simulink model "ai_optimal_path_depth_v2_4_g100"  (R2020a)
settings: Solver=FixedStepDiscrete  StartTime=0.0  StopTime=inf  FixedStep=0.2  RelTol=1e-3  EnableMultiTasking=on
model workspace (MAT data in the model file):
  SL_ROS_VariableLengthArrays_MaxSizes : object (value not decoded)
undefined symbols (not defined in the file): Data, Data_SL_Info
libraries: robotlib x33
(part 2 of 2)

== matlab function ai_optimal_path_depth_v2_4_g100/MATLAB Function ==
  data: current_pos input; point input; distance input; bboxes_front_raw input; bboxes_back_raw input; bboxes_left_raw input; bboxes_right_raw input; openpoint_front output; image_size input; image_grid input; openpoint_back output; openpoint_left output; openpoint_right output; count output; obstacle_check output
function [openpoint_front,openpoint_back,openpoint_left,openpoint_right,count,obstacle_check] = fcn(current_pos,point,distance,bboxes_front_raw,bboxes_back_raw,bboxes_left_raw,bboxes_right_raw,image_size,image_grid)
% function [distance_ref_front,distance_ref_back,distance_ref_left,distance_ref_right] = fcn(point,I_front_rgb,I_back_rgb,I_left_rgb,I_right_rgb,bboxes_front_raw,bboxes_back_raw,bboxes_left_raw,bboxes_right_raw)
% image_grid = 0.05;

% pos_x = current_pos(1);
% pos_y = current_pos(2);
% pos_z = current_pos(3);
% pos_x = current_pos.Poses(end).Pose.Position.X;
% pos_y = current_pos.Poses(end).Pose.Position.Y;
% pos_z = current_pos.Poses(end).Pose.Position.Z;

pos_x = current_pos.Pose.Pose.Position.X;
pos_y = current_pos.Pose.Pose.Position.Y;
pos_z = current_pos.Pose.Pose.Position.Z;
% image_size = 500;
% image_size = I_front_rgb(:,:,1);
% image_size = I_back_rgb(:,:,1);
% image_size = I_left_rgb(:,:,1);
% image_size = I_right_rgb(:,:,1);

openpoint_front = nan(5,6);
openpoint_back = nan(5,6);
openpoint_left = nan(5,6);
openpoint_right = nan(5,6);
count = zeros(5,4);
obstacle_check = zeros(5,4);
thickness = distance/2;
% thickness = 2;
obstacle_safety = 0.3;

% bboxes_front = int16(bboxes_front_raw);
% bboxes_back = int16(bboxes_back_raw);
% bboxes_left = int16(bboxes_left_raw);
% bboxes_right = int16(bboxes_right_raw);
% bboxes_front = reshape(int16(bboxes_front_raw),[5, 4]);
% bboxes_back = reshape(int16(bboxes_back_raw),[5, 4]);
% bboxes_left = reshape(int16(bboxes_left_raw),[5, 4]);
% bboxes_right = reshape(int16(bboxes_right_raw),[5, 4]);

bboxes_front = nan(5,4);
bboxes_back = nan(5,4);
bboxes_left = nan(5,4);
bboxes_right = nan(5,4);
for ttt = 1:4
    for sss = 1:5
        bboxes_front(sss,ttt) = int16(bboxes_front_raw(5*(ttt-1)+sss));
        bboxes_back(sss,ttt) = int16(bboxes_back_raw(5*(ttt-1)+sss));
        bboxes_left(sss,ttt) = int16(bboxes_left_raw(5*(ttt-1)+sss));
        bboxes_right(sss,ttt) = int16(bboxes_right_raw(5*(ttt-1)+sss));
    end
end
        
% distance_ref_front=[];
% distance_ref_back=[];
% distance_ref_left=[];
% distance_ref_right=[];

distance_ref_front=nan(5,1);
distance_ref_back=nan(5,1);
distance_ref_left=nan(5,1);
distance_ref_right=nan(5,1);

% aaa=1;
% if ~isempty(bboxes_front)
if ~sum(bboxes_front)==0
    for aaa = 1:numel(nonzeros(bboxes_front))/4
        if (bboxes_front(aaa,1)+bboxes_front(aaa,3)/2) >= (image_size)/2
            distance_ref_front(aaa) = bboxes_front(aaa,1)+bboxes_front(aaa,3);
        else
            distance_ref_front(aaa) = bboxes_front(aaa,1);
        end
    end
    distance_ref_front= -(distance_ref_front - (image_size)/2)*image_grid;           % 醫뚰몴媛?(m)
end

% if ~isempty(bboxes_back)
if ~sum(bboxes_back)==0
    for aaa = 1:numel(nonzeros(bboxes_back))/4
        if (bboxes_back(aaa,1)+bboxes_back(aaa,3)/2) >= (image_size)/2
            distance_ref_back(aaa) = bboxes_back(aaa,1)+bboxes_back(aaa,3);
        else
            distance_ref_back(aaa) = bboxes_back(aaa,1);
        end
    end
    distance_ref_back= -(distance_ref_back - (image_size)/2)*image_grid;              % 醫뚰몴媛?(m)
end

% if ~isempty(bboxes_left)
if ~sum(bboxes_left)==0
    for aaa = 1:numel(nonzeros(bboxes_left))/4
        if (bboxes_left(aaa,1)+bboxes_left(aaa,3)/2) >= (image_size)/2
            distance_ref_left(aaa) = bboxes_left(aaa,1)+bboxes_left(aaa,3);
        else
            distance_ref_left(aaa) = bboxes_left(aaa,1);
        end
    end
    distance_ref_left= (distance_ref_left - (image_size)/2)*image_grid;              % 醫뚰몴媛?(m)
end

% if ~isempty(bboxes_right)
if ~sum(bboxes_right)==0
    for aaa = 1:numel(nonzeros(bboxes_right))/4
        if (bboxes_right(aaa,1)+bboxes_right(aaa,3)/2) >= (image_size)/2
            distance_ref_right(aaa) = bboxes_right(aaa,1)+bboxes_right(aaa,3);
        else
            distance_ref_right(aaa) = bboxes_right(aaa,1);
        end
    end
    distance_ref_right= (distance_ref_right - (image_size)/2)*image_grid;            % 醫뚰몴媛?(m)
end

% scale = 5;
% scale = 20;
scale = 1/image_grid;
distance_fb_max=-ones(length(distance_ref_front),1)*image_grid*(image_size)/2;
distance_fb_min=ones(length(distance_ref_back),1)*image_grid*(image_size)/2;
distance_lr_max=-ones(length(distance_ref_left),1)*image_grid*(image_size)/2;
distance_lr_min=ones(length(distance_ref_right),1)*image_grid*(image_size)/2;

% distance_fb_max=ones(5,1)*distance;
% distance_fb_min=-ones(5,1)*distance;
% distance_lr_max=ones(5,1)*distance;
% distance_lr_min=-ones(5,1)*distance;
    
for bbb=1:length(point)
    %     if ~isempty(distance_ref_front)
    for aaa = 1:length(distance_ref_front)
        if ~isnan(distance_ref_front(aaa))
            if point(bbb,2)>=(distance_ref_front(aaa)-image_grid*scale) && point(bbb,2)<=(distance_ref_front(aaa)+image_grid*scale)
                if point(bbb,1) > distance_fb_max(aaa)
                    distance_fb_max(aaa) = point(bbb,1);
                end
            end
        end
    end
    %     if ~isempty(distance_ref_back)
    for aaa = 1:length(distance_ref_back)
        if ~isnan(distance_ref_back(aaa))
            if point(bbb,2)>=(distance_ref_back(aaa)-image_grid*scale) && point(bbb,2)<=(distance_ref_back(aaa)+image_grid*scale)
                if point(bbb,1) < distance_fb_min(aaa)
                    distance_fb_min(aaa) = point(bbb,1);
                end
            end
        end
    end
    %     if ~isempty(distance_ref_left)
    for aaa = 1:length(distance_ref_left)
        if ~isnan(distance_ref_left(aaa))
            if point(bbb,1)>=(distance_ref_left(aaa)-image_grid*scale) && point(bbb,1)<=(distance_ref_left(aaa)+image_grid*scale)
                if point(bbb,2) > distance_lr_max(aaa)
                    distance_lr_max(aaa) = point(bbb,2);
                end
            end
        end
    end
    %     if ~isempty(distance_ref_right)
    for aaa = 1:length(distance_ref_right)
        if ~isnan(distance_ref_right(aaa))
            if point(bbb,1)>=(distance_ref_right(aaa)-image_grid*scale) && point(bbb,1)<=(distance_ref_right(aaa)+image_grid*scale)
                if point(bbb,2) < distance_lr_min(aaa)
                    distance_lr_min(aaa) = point(bbb,2);
                end
            end
        end
    end
end
bboxes_transformed_front = -(double(bboxes_front)-[ones(5,1)*(image_size)/2, ones(5,1)*(image_size)/2, zeros(5,1), zeros(5,1)])*image_grid;
bboxes_transformed_back = -(double(bboxes_back)-[ones(5,1)*(image_size)/2, ones(5,1)*(image_size)/2, zeros(5,1), zeros(5,1)])*image_grid;
bboxes_transformed_left = (double(bboxes_left)-[ones(5,1)*(image_size)/2, ones(5,1)*(image_size)/2, zeros(5,1), zeros(5,1)]).*[ones(5,1), -ones(5,1), ones(5,1), -ones(5,1)]*image_grid;
bboxes_transformed_right = (double(bboxes_right)-[ones(5,1)*(image_size)/2, ones(5,1)*(image_size)/2, zeros(5,1), zeros(5,1)]).*[ones(5,1), -ones(5,1), ones(5,1), -ones(5,1)]*image_grid;

%(x,y,z,length,width,height)
% openpoint_front = [distance_fb_max-thickness/2,bboxes_transformed_front(:,1)+bboxes_transformed_front(:,3)/2,bboxes_transformed_front(:,2)+bboxes_transformed_front(:,4)/2,thickness*ones(length(distance_fb_max),1),abs(bboxes_transformed_front(:,3)),abs(bboxes_transformed_front(:,4))];                      
% openpoint_back = [distance_fb_min+thickness/2,bboxes_transformed_back(:,1)+bboxes_transformed_back(:,3)/2,bboxes_transformed_back(:,2)+bboxes_transformed_back(:,4)/2,thickness*ones(length(distance_fb_min),1),abs(bboxes_transformed_back(:,3)),abs(bboxes_transformed_back(:,4))];
% openpoint_left = [bboxes_transformed_left(:,1)+bboxes_transformed_left(:,3)/2 , distance_lr_max-thickness/2 , bboxes_transformed_left(:,2)+bboxes_transformed_left(:,4)/2,abs(bboxes_transformed_left(:,3)),thickness*ones(length(distance_lr_max),1),abs(bboxes_transformed_left(:,4))];
% openpoint_right = [bboxes_transformed_right(:,1)+bboxes_transformed_right(:,3)/2 , distance_lr_min+thickness/2 , bboxes_transformed_right(:,2)+bboxes_transformed_right(:,4)/2,abs(bboxes_transformed_right(:,3)),thickness*ones(length(distance_lr_min),1),abs(bboxes_transformed_right(:,4))];

for aaa = 1 : 5
    if ~(distance_fb_max(aaa) == -image_grid*image_size/2)
        openpoint_front(aaa,:) = [distance_fb_max(aaa)-thickness/2 , bboxes_transformed_front(aaa,1)+bboxes_transformed_front(aaa,3)/2+pos_y , bboxes_transformed_front(aaa,2)+bboxes_transformed_front(aaa,4)/2+pos_z , thickness , abs(bboxes_transformed_front(aaa,3)) , abs(bboxes_transformed_front(aaa,4))];
%         openpoint_front(aaa,:) = [distance_fb_max(aaa)-thickness/2+pos_x , bboxes_transformed_front(aaa,1)+bboxes_transformed_front(aaa,3)/2+pos_y , bboxes_transformed_front(aaa,2)+bboxes_transformed_front(aaa,4)/2+pos_z , thickness , abs(bboxes_transformed_front(aaa,3)) , abs(bboxes_transformed_front(aaa,4))];
    end
    if ~(distance_fb_min(aaa) == image_grid*image_size/2)
        openpoint_back(aaa,:) = [distance_fb_min(aaa)+thickness/2 , bboxes_transformed_back(aaa,1)+bboxes_transformed_back(aaa,3)/2+pos_y , bboxes_transformed_back(aaa,2)+bboxes_transformed_back(aaa,4)/2+pos_z , thickness , abs(bboxes_transformed_back(aaa,3)) , abs(bboxes_transformed_back(aaa,4))];
%         openpoint_back(aaa,:) = [distance_fb_min(aaa)+thickness/2+pos_x , bboxes_transformed_back(aaa,1)+bboxes_transformed_back(aaa,3)/2+pos_y , bboxes_transformed_back(aaa,2)+bboxes_transformed_back(aaa,4)/2+pos_z , thickness , abs(bboxes_transformed_back(aaa,3)) , abs(bboxes_transformed_back(aaa,4))];
    end
    if ~(distance_lr_max(aaa) == -image_grid*image_size/2)
        openpoint_left(aaa,:) = [bboxes_transformed_left(aaa,1)+bboxes_transformed_left(aaa,3)/2+pos_x , distance_lr_max(aaa)-thickness/2 , bboxes_transformed_left(aaa,2)+bboxes_transformed_left(aaa,4)/2+pos_z , abs(bboxes_transformed_left(aaa,3)) , thickness , abs(bboxes_transformed_left(aaa,4))];
%         openpoint_left(aaa,:) = [bboxes_transformed_left(aaa,1)+bboxes_transformed_left(aaa,3)/2+pos_x , distance_lr_max(aaa)-thickness/2+pos_y , bboxes_transformed_left(aaa,2)+bboxes_transformed_left(aaa,4)/2+pos_z , abs(bboxes_transformed_left(aaa,3)) , thickness , abs(bboxes_transformed_left(aaa,4))];
    end
    if ~(distance_lr_min(aaa) == image_grid*image_size/2)
        openpoint_right(aaa,:) = [bboxes_transformed_right(aaa,1)+bboxes_transformed_right(aaa,3)/2+pos_x , distance_lr_min(aaa)+thickness/2 , bboxes_transformed_right(aaa,2)+bboxes_transformed_right(aaa,4)/2+pos_z , abs(bboxes_transformed_right(aaa,3)) , thickness , abs(bboxes_transformed_right(aaa,4))];
%         openpoint_right(aaa,:) = [bboxes_transformed_right(aaa,1)+bboxes_transformed_right(aaa,3)/2+pos_x , distance_lr_min(aaa)+thickness/2+pos_y , bboxes_transformed_right(aaa,2)+bboxes_transformed_right(aaa,4)/2+pos_z , abs(bboxes_transformed_right(aaa,3)) , thickness , abs(bboxes_transformed_right(aaa,4))];
    end
end

for aaa = 1:5
    count_front = 0;
    count_back = 0;
    count_left = 0;
    count_right = 0;
    obstacle_check_front = 0;
    obstacle_check_back = 0;
    obstacle_check_left = 0;
    obstacle_check_right = 0;
    for bbb = 1:length(point)
        if ((point(bbb,1) > openpoint_front(aaa,1)-thickness/10) && (point(bbb,1) < openpoint_front(aaa,1)+thickness/10)) && (point(bbb,2) > openpoint_front(aaa,2)-thickness/10) && (point(bbb,2) < openpoint_front(aaa,2)+thickness/10)
%         if ((point(bbb,1) > openpoint_front(aaa,1)-thickness/2-thickness/10) && (point(bbb,1) < openpoint_front(aaa,1)-thickness/2+thickness/10)) && (point(bbb,2) > openpoint_front(aaa,2)-thickness/10) && (point(bbb,2) < openpoint_front(aaa,2)+thickness/10)
            count_front = count_front+1;
        end
        if ((point(bbb,1) > openpoint_back(aaa,1)-thickness/10) && (point(bbb,1) < openpoint_back(aaa,1)+thickness/10)) && (point(bbb,2) > openpoint_back(aaa,2)-thickness/10) && (point(bbb,2) < openpoint_back(aaa,2)+thickness/10)
%         if ((point(bbb,1) > openpoint_back(aaa,1)+thickness/2-thickness/10) && (point(bbb,1) < openpoint_back(aaa,1)+thickness/2+thickness/10)) && (point(bbb,2) > openpoint_back(aaa,2)-thickness/10) && (point(bbb,2) < openpoint_back(aaa,2)+thickness/10)
            count_back = count_back+1;
        end
        if ((point(bbb,1) > openpoint_left(aaa,1)-thickness/10) && (point(bbb,1) < openpoint_left(aaa,1)+thickness/10)) && (point(bbb,2) > openpoint_left(aaa,2)-thickness/10) && (point(bbb,2) < openpoint_left(aaa,2)+thickness/10)
%         if ((point(bbb,1) > openpoint_left(aaa,1)-thickness/10) && (point(bbb,1) < openpoint_left(aaa,1)+thickness/10)) && (point(bbb,2) > openpoint_left(aaa,2)-thickness/2-thickness/10) && (point(bbb,2) < openpoint_left(aaa,2)-thickness/2+thickness/10)
            count_left = count_left+1;
        end
        if ((point(bbb,1) > openpoint_right(aaa,1)-thickness/10) && (point(bbb,1) < openpoint_right(aaa,1)+thickness/10)) && (point(bbb,2) > openpoint_right(aaa,2)-thickness/10) && (point(bbb,2) < openpoint_right(aaa,2)+thickness/10)
%         if ((point(bbb,1) > openpoint_right(aaa,1)-thickness/10) && (point(bbb,1) < openpoint_right(aaa,1)+thickness/10)) && (point(bbb,2) > openpoint_right(aaa,2)+thickness/2-thickness/10) && (point(bbb,2) < openpoint_right(aaa,2)+thickness/2+thickness/10)
            count_right= count_right+1;
        end
        
        if ((point(bbb,1) > openpoint_front(aaa,1)-obstacle_safety) && (point(bbb,1) < openpoint_front(aaa,1)+obstacle_safety)) && ((point(bbb,2) > openpoint_front(aaa,2)-obstacle_safety) && (point(bbb,2) < openpoint_front(aaa,2)+obstacle_safety)) && ((point(bbb,3) > openpoint_front(aaa,3)-obstacle_safety) && (point(bbb,3) < openpoint_front(aaa,3)+obstacle_safety))
            obstacle_check_front = obstacle_check_front+1;
        end
        if ((point(bbb,1) > openpoint_back(aaa,1)-obstacle_safety) && (point(bbb,1) < openpoint_back(aaa,1)+obstacle_safety)) && ((point(bbb,2) > openpoint_back(aaa,2)-obstacle_safety) && (point(bbb,2) < openpoint_back(aaa,2)+obstacle_safety)) && ((point(bbb,3) > openpoint_back(aaa,3)-obstacle_safety) && (point(bbb,3) < openpoint_back(aaa,3)+obstacle_safety))
            obstacle_check_back = obstacle_check_back+1;
        end
        if ((point(bbb,1) > openpoint_left(aaa,1)-obstacle_safety) && (point(bbb,1) < openpoint_left(aaa,1)+obstacle_safety)) && ((point(bbb,2) > openpoint_left(aaa,2)-obstacle_safety) && (point(bbb,2) < openpoint_left(aaa,2)+obstacle_safety)) && ((point(bbb,3) > openpoint_left(aaa,3)-obstacle_safety) && (point(bbb,3) < openpoint_left(aaa,3)+obstacle_safety))
            obstacle_check_left = obstacle_check_left+1;
        end
        if ((point(bbb,1) > openpoint_right(aaa,1)-obstacle_safety) && (point(bbb,1) < openpoint_right(aaa,1)+obstacle_safety)) && ((point(bbb,2) > openpoint_right(aaa,2)-obstacle_safety) && (point(bbb,2) < openpoint_right(aaa,2)+obstacle_safety)) && ((point(bbb,3) > openpoint_right(aaa,3)-obstacle_safety) && (point(bbb,3) < openpoint_right(aaa,3)+obstacle_safety))
            obstacle_check_right= obstacle_check_right+1;
        end
        
    end
    %유효성 체크
    count(aaa,:) = [count_front, count_back, count_left, count_right];
    obstacle_check(aaa,:) = [obstacle_check_front, obstacle_check_back, obstacle_check_left, obstacle_check_right];
    if count_front < 2 || obstacle_check_front > 0
%     if obstacle_check_front > 0
        openpoint_front(aaa,:) = nan(1,6);
    end
    if count_back< 2 || obstacle_check_back > 0
%     if obstacle_check_back > 0
        openpoint_back(aaa,:) = nan(1,6);
    end
    if count_left< 2 || obstacle_check_left > 0
%     if obstacle_check_left > 0
        openpoint_left(aaa,:) = nan(1,6);
    end
    if count_right< 2 || obstacle_check_right > 0
%     if obstacle_check_right > 0
        openpoint_right(aaa,:) = nan(1,6);
    end
end

== matlab function ai_optimal_path_depth_v2_4_g100/MATLAB Function4 ==
  data: pos_cur input; distance input; waypoint_gen output; pos_init input; openpoint_front input; openpoint_back input; openpoint_left input; openpoint_right input; pos_explor_grid output
function [waypoint_gen,pos_explor_grid] = fcn(pos_cur,distance,pos_init,openpoint_front,openpoint_back,openpoint_left,openpoint_right)

persistent explor_grid

if isempty(explor_grid)
    explor_grid = zeros(50,50,10);
end

% pos_x = current_pos(1);
% pos_y = current_pos(2);
% pos_z = current_pos(3);
% pos_x = pos_cur.Poses(end).Pose.Position.X;
% pos_y = pos_cur.Poses(end).Pose.Position.Y;
% pos_z = pos_cur.Poses(end).Pose.Position.Z;

pos_x = pos_cur.Pose.Pose.Position.X;
pos_y = pos_cur.Pose.Pose.Position.Y;
pos_z = pos_cur.Pose.Pose.Position.Z;

% grid_explor_size = 4;
% grid_explor_size = distance/2;
grid_explor_size = distance/4;
grid_size = 0.1;
explor_map_init = [25, 25, 5];
pos_explor_grid = int32([pos_x/grid_explor_size+explor_map_init(1), pos_y/grid_explor_size+explor_map_init(2) , pos_z/grid_explor_size+explor_map_init(3)]);

explor_grid(pos_explor_grid(1),pos_explor_grid(2),pos_explor_grid(3))=1;



for abc=1:numel(openpoint_front)/6
    if ~isnan(openpoint_front(abc,1)) && ~isnan(openpoint_front(abc,2)) && ~isnan(openpoint_front(abc,3))
        if explor_grid(int16(openpoint_front(abc,1)/grid_explor_size+explor_map_init(1)),int16(openpoint_front(abc,2)/grid_explor_size+explor_map_init(2)),int16(openpoint_front(abc,3)/grid_explor_size+explor_map_init(3))) == 1
            openpoint_front(abc,:) = nan(1,6);
        end
    end
end
for abc=1:numel(openpoint_back)/6
    if ~isnan(openpoint_back(abc,1)) && ~isnan(openpoint_back(abc,2)) && ~isnan(openpoint_back(abc,3))
        if explor_grid(int16(openpoint_back(abc,1)/grid_explor_size+explor_map_init(1)),int16(openpoint_back(abc,2)/grid_explor_size+explor_map_init(2)),int16(openpoint_back(abc,3)/grid_explor_size+explor_map_init(3))) == 1
            openpoint_back(abc,:) = nan(1,6);
        end
    end
end
for abc=1:numel(openpoint_left)/6
    if ~isnan(openpoint_left(abc,1)) && ~isnan(openpoint_left(abc,2)) && ~isnan(openpoint_left(abc,3))
        if explor_grid(int16(openpoint_left(abc,1)/grid_explor_size+explor_map_init(1)),int16(openpoint_left(abc,2)/grid_explor_size+explor_map_init(2)),int16(openpoint_left(abc,3)/grid_explor_size+explor_map_init(3))) == 1
            openpoint_left(abc,:) = nan(1,6);
        end
    end
end
for abc=1:numel(openpoint_right)/6
    if ~isnan(openpoint_right(abc,1)) && ~isnan(openpoint_right(abc,2)) && ~isnan(openpoint_right(abc,3))
        if explor_grid(int16(openpoint_right(abc,1)/grid_explor_size+explor_map_init(1)),int16(openpoint_right(abc,2)/grid_explor_size+explor_map_init(2)),int16(openpoint_right(abc,3)/grid_explor_size+explor_map_init(3))) == 1
            openpoint_right(abc,:) = nan(1,6);
        end
    end
end



openpoint_front_grid = int16(openpoint_front/grid_size);
openpoint_back_grid = int16(openpoint_back/grid_size);
openpoint_left_grid = int16(openpoint_left/grid_size);
openpoint_right_grid = int16(openpoint_right/grid_size);



waypoint_gen_front = nan(5,3);
waypoint_gen_back = nan(5,3);
waypoint_gen_left = nan(5,3);
waypoint_gen_right = nan(5,3);

for aaa = 1:5
    if ~isnan(openpoint_front(aaa,1))
        waypoint_gen_front(aaa,:) = [openpoint_front_grid(aaa,1)+int16(pos_init(1)), openpoint_front_grid(aaa,2)+int16(pos_init(2)), openpoint_front_grid(aaa,3)+int16(pos_init(3))];
    end
    if ~isnan(openpoint_back(aaa,1))
        waypoint_gen_back(aaa,:) = [openpoint_back_grid(aaa,1)+int16(pos_init(1)), openpoint_back_grid(aaa,2)+int16(pos_init(2)), openpoint_back_grid(aaa,3)+int16(pos_init(3))];
    end
    if ~isnan(openpoint_left(aaa,1))
        waypoint_gen_left(aaa,:) = [openpoint_left_grid(aaa,1)+int16(pos_init(1)), openpoint_left_grid(aaa,2)+int16(pos_init(2)), openpoint_left_grid(aaa,3)+int16(pos_init(3))];
    end
    if ~isnan(openpoint_right(aaa,1))
        waypoint_gen_right(aaa,:) = [openpoint_right_grid(aaa,1)+int16(pos_init(1)), openpoint_right_grid(aaa,2)+int16(pos_init(2)), openpoint_right_grid(aaa,3)+int16(pos_init(3))];
    end
end



waypoint_gen = [waypoint_gen_front;waypoint_gen_back;waypoint_gen_left;waypoint_gen_right];

%%%%%%%%%%%%%%%%%%%%%%%%%%%%%%%%%%%% for back safety
for lll = 1:numel(waypoint_gen)/3
    if waypoint_gen(lll,1)<-0.5
        waypoint_gen(lll,:) = nan(1,3);
    end
end

== matlab function ai_optimal_path_depth_v2_4_g100/MATLAB Function5 ==
  data: data input size=[40 3]; test output size=[1 128]; SL output
function [test,SL]   = func(data)

% test = single(nan(1,128));

test = single([data(:,1)', nan(1,88)]);
% for i = 1:length(data)
%     test(i) = single(data(i));
% end

SL = uint32(length(data(:,1)));


end

== matlab function ai_optimal_path_depth_v2_4_g100/MATLAB Function6 ==
  data: data input size=[20 1]; test output size=[1 128]; SL output
function [test,SL]   = func(data)

% test = single(nan(1,128));

test = single([data(:,1)', nan(1,108)]);
% for i = 1:length(data)
%     test(i) = single(data(i));
% end

SL = uint32(length(data(:,1)));


end
